simulink model "ThermalModel"  (R2021a)
settings: Solver=FixedStepAuto  StartTime=0.0  StopTime=28600  FixedStep=0.2  RelTol=1e-3
InitFcn:
  | %StartUp_VariableDeclaration;
undefined symbols (not defined in the file or in its folder): AxAlpha_Bottoms_Ambient, AxAlpha_Column_Ambient, AxAlpha_Head_Ambient, AxAlpha_Heater_Ambient, AxAlpha_Heater_Bottoms_Off, AxAlpha_Heater_Bottoms_On, AxAlpha_Heater_Inner_Outer, AxAlpha_Template, M_Water_Template, MxC_Bottoms, MxC_Column, MxC_Head, MxC_Heater_Inner, MxC_Heater_Outer, MxC_Template, T_init_Bottoms, T_init_Column, T_init_Head, T_init_Heater, T_init_Template, Temp_Water_Initial_Template
settings Model: OrderedModelArguments=off  Creator=Reinpold  LastModifiedBy=Reinpold

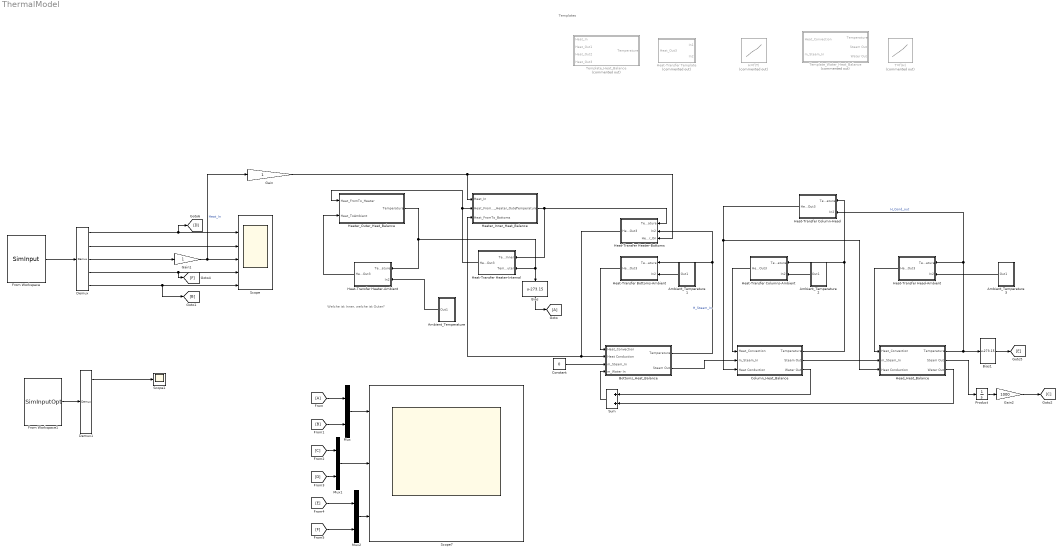
== system ThermalModel ==
  note: Welche ist Inner, welche ist Outer?
  note: Templates
  Ambient_Temperature : Subsystem
  Ambient_Temperature1 : Subsystem
  Ambient_Temperature2 : Subsystem
  Ambient_Temperature3 : Subsystem
  Bias : Bias  Bias=-273.15
  Bias1 : Bias  Bias=-273.15
  Bottoms_Heat_Balance : Subsystem
  Column_Heat_Balance : Subsystem
  Constant : Constant  Value=0
  Demux : Demux  Outputs=5
  Demux1 : Demux
  From Workspace : FromWorkspace  VariableName=SimInput
  From Workspace1 : FromWorkspace  VariableName=SimInputOpt  Interpolate=off  OutputAfterFinalValue=Holding final value
  Gain : Gain
  Gain1 : Gain
  Gain2 : Gain  Gain=1000
  H=f(T) : Lookup_n-D  Commented=on  NumberOfTableDimensions=1  BreakpointsForDimension1=|  Table=[0.10319804238124, 414.95098616583, 2675.58417423615, 2822.05078480503]  InternalRulePriority=Speed  RndMeth=Simplest  InputSameDT=on
      | [273.16, 372.15, 373.15, 446.15
      | ]
  Head_Heat_Balance : Subsystem
  Heat-Transfer Bottoms-Ambient : Subsystem
  Heat-Transfer Column-Head : Subsystem
  Heat-Transfer Columns-Ambient : Subsystem
  Heat-Transfer Head-Ambient : Subsystem
  Heat-Transfer Heater-Ambient : Subsystem
  Heat-Transfer Heater-Bottoms : Subsystem
  Heat-Transfer Heater-Internal : Subsystem
  Heat-Transfer Template : Subsystem  Commented=on
  Heater_Inner_Heat_Balance : Subsystem
  Heater_Outer_Heat_Balance : Subsystem
  Mux : Mux  Inputs=2
  Mux1 : Mux  Inputs=2
  Mux2 : Mux  Inputs=2
  Product : Integrator
  Scope : Scope  NumInputPorts=6
  Scope1 : Scope
  Scope7 : Scope  NumInputPorts=3
  Sum : Sum
  T=f(H) : Lookup_n-D  Commented=on  NumberOfTableDimensions=1  BreakpointsForDimension1=[0.10319804238124, 414.95098616583, 2675.58417423615, 2822.05078480503]  Table=[273.16, 372.15, 373.15, 446.15]  InternalRulePriority=Speed  RndMeth=Simplest  InputSameDT=on
  Template_Heat_Balance : Subsystem  Commented=on
  Template_Water_Heat_Balance : Subsystem  Commented=on
  wires:
  Gain1/1 -> Gain/1, Scope/4  "Heat_In"
  Ambient_Temperature/1(Out1) -> Heat-Transfer Heater-Ambient/2(In2)
  Heat-Transfer Heater-Ambient/1(Heat_Out3) -> Heater_Outer_Heat_Balance/2(Heat_ToAmbient)
  Heat-Transfer Heater-Bottoms/1(Heat_Out3) -> Bottoms_Heat_Balance/2(Heat Conduction), Heater_Inner_Heat_Balance/3(Heat_FromTo_Bottoms)
  Ambient_Temperature1/1(Out1) -> Heat-Transfer Bottoms-Ambient/2(In2)
  Heat-Transfer Bottoms-Ambient/1(Heat_Out3) -> Bottoms_Heat_Balance/1(Heat_Convection)
  Heat-Transfer Columns-Ambient/1(Heat_Out3) -> Column_Heat_Balance/1(Heat_Convection)
  Ambient_Temperature2/1(Out1) -> Heat-Transfer Columns-Ambient/2(In2)
  Heat-Transfer Head-Ambient/1(Heat_Out3) -> Head_Heat_Balance/1(Heat_Convection)
  Ambient_Temperature3/1(Out1) -> Heat-Transfer Head-Ambient/2(In2)
  Constant/1 -> Bottoms_Heat_Balance/3(m_Steam_In)
  Column_Heat_Balance/2(Steam Out) -> Head_Heat_Balance/2(m_Steam_In)
  Bottoms_Heat_Balance/2(Steam Out) -> Column_Heat_Balance/2(m_Steam_In)
  Product/1 -> Gain2/1
  Sum/1 -> Bottoms_Heat_Balance/4(m_Water In)
  Demux/2 -> Scope/3
  Demux/5 -> [B], Scope/6
  Bias1/1 -> [E]
  Column_Heat_Balance/3(Water Out) -> Sum/1
  Head_Heat_Balance/3(Water Out) -> Sum/2
  Head_Heat_Balance/2(Steam Out) -> Product/1
  From Workspace/1 -> Demux/1
  Gain2/1 -> [C]
  Heat-Transfer Column-Head/1(Heat_Out3) -> Head_Heat_Balance/3(Heat Conduction), Column_Heat_Balance/3(Heat Conduction)
  Column_Heat_Balance/1(Temperature) -> Heat-Transfer Columns-Ambient/1(Temperature), Heat-Transfer Column-Head/1(Temperature)
  Head_Heat_Balance/1(Temperature) -> Bias1/1, Heat-Transfer Column-Head/2(In2), Heat-Transfer Head-Ambient/1(Temperature)  "H_Cond_out"
  Heater_Inner_Heat_Balance/1(Temperature) -> Heat-Transfer Heater-Internal/1(Temperature_Inner), Heat-Transfer Heater-Bottoms/1(Temperature)
  Bottoms_Heat_Balance/1(Temperature) -> Heat-Transfer Heater-Bottoms/2(In2), Heat-Transfer Bottoms-Ambient/1(Temperature)  "H_Steam_In"
  Heater_Outer_Heat_Balance/1(Temperature) -> Bias/1, Heat-Transfer Heater-Internal/2(Temperature_Outer), Heat-Transfer Heater-Ambient/1(Temperature)
  Heat-Transfer Heater-Internal/1(Heat_Out3) -> Heater_Inner_Heat_Balance/2(Heat_FromTo_Heater_Outer), Heater_Outer_Heat_Balance/1(Heat_FromTo_Heater)
  [A] -> Mux/1
  [B] -> Mux/2
  [C] -> Mux1/1
  [D] -> Mux1/2
  [E] -> Mux2/1
  [F] -> Mux2/2
  Mux/1 -> Scope7/1
  Mux1/1 -> Scope7/2
  Mux2/1 -> Scope7/3
  Gain/1 -> Heat-Transfer Heater-Bottoms/3(Heater_On), Heater_Inner_Heat_Balance/1(Heat_In)
  Bias/1 -> [A]
  From Workspace1/1 -> Demux1/1
  Demux/1 -> Scope/2, [D]
  Demux/4 -> [F], Scope/5
  Demux/3 -> Gain1/1
  Demux1/1 -> Scope1/1

== system ThermalModel/Ambient_Temperature ==
  1-D Lookup Table : Lookup_n-D  NumberOfTableDimensions=1  BreakpointsForDimension1=[0,90*60,180*60,270*60,360*60]  Table=[21,23,23.5,24,24]  InternalRulePriority=Speed  RndMeth=Simplest  InputSameDT=on
  Bias2 : Bias  Bias=273.15
  Clock : Clock
  Out1 : Outport
  wires:
  1-D Lookup Table/1 -> Bias2/1
  Bias2/1 -> Out1/1
  Clock/1 -> 1-D Lookup Table/1

== system ThermalModel/Ambient_Temperature1 ==
  1-D Lookup Table : Lookup_n-D  NumberOfTableDimensions=1  BreakpointsForDimension1=[0,90*60,180*60,270*60,360*60]  Table=[21,23,23.5,24,24]  InternalRulePriority=Speed  RndMeth=Simplest  InputSameDT=on
  Bias2 : Bias  Bias=273.15
  Clock : Clock
  Out1 : Outport
  wires:
  1-D Lookup Table/1 -> Bias2/1
  Bias2/1 -> Out1/1
  Clock/1 -> 1-D Lookup Table/1

== system ThermalModel/Ambient_Temperature2 ==
  1-D Lookup Table : Lookup_n-D  NumberOfTableDimensions=1  BreakpointsForDimension1=[0,90*60,180*60,270*60,360*60]  Table=[21,23,23.5,24,24]  InternalRulePriority=Speed  RndMeth=Simplest  InputSameDT=on
  Bias2 : Bias  Bias=273.15
  Clock : Clock
  Out1 : Outport
  wires:
  1-D Lookup Table/1 -> Bias2/1
  Bias2/1 -> Out1/1
  Clock/1 -> 1-D Lookup Table/1

== system ThermalModel/Ambient_Temperature3 ==
  1-D Lookup Table : Lookup_n-D  NumberOfTableDimensions=1  BreakpointsForDimension1=[0,90*60,180*60,270*60,360*60]  Table=[21,23,23.5,24,24]  InternalRulePriority=Speed  RndMeth=Simplest  InputSameDT=on
  Bias2 : Bias  Bias=273.15
  Clock : Clock
  Out1 : Outport
  wires:
  1-D Lookup Table/1 -> Bias2/1
  Bias2/1 -> Out1/1
  Clock/1 -> 1-D Lookup Table/1

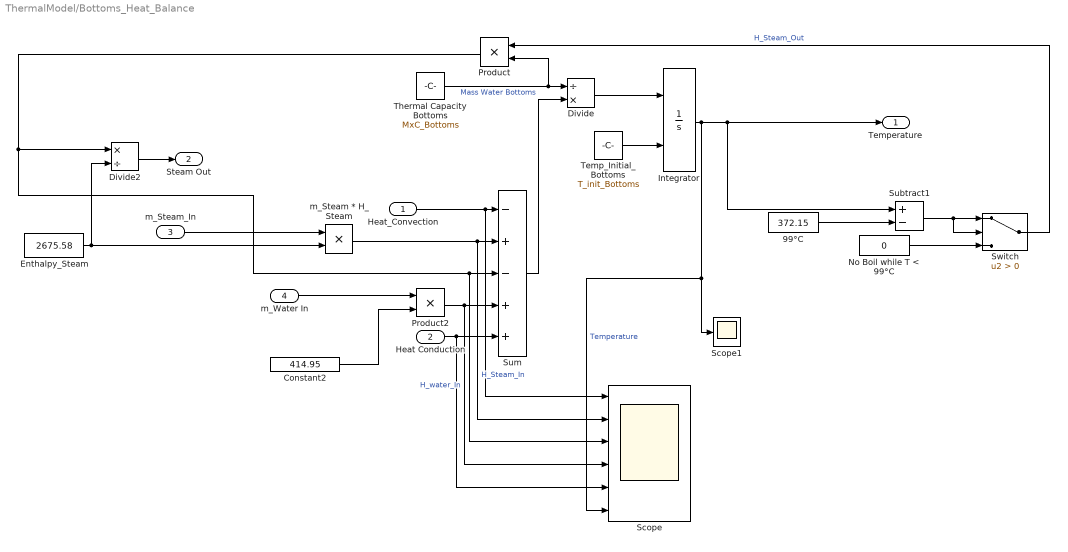
== system ThermalModel/Bottoms_Heat_Balance ==
  Heat_Convection : Inport
  Heat Conduction : Inport  Port=2
  m_Steam_In : Inport  Port=3
  m_Water In : Inport  Port=4
  " 99°C" : Constant  Value=372.15
  Constant2 : Constant  Value=414.95
  Divide : Product  Inputs=/*
  Divide2 : Product  Inputs=*/
  Enthalpy_Steam : Constant  Value=2675.58
  Integrator : Integrator  InitialConditionSource=external  UpperSaturationLimit=100
  No Boil while T < 99°C : Constant  Value=0
  Product : Product
  Product2 : Product
  Scope : Scope  NumInputPorts=6
  Scope1 : Scope
  Subtract1 : Sum  Inputs=+-
  Sum : Sum  Inputs=-+-++
  Switch : Switch  Criteria=u2 > Threshold
  Temp_Initial_Bottoms : Constant  Value=T_init_Bottoms
  Thermal Capacity Bottoms : Constant  Value=MxC_Bottoms
  m_Steam * H_Steam : Product
  Temperature : Outport
  Steam Out : Outport  Port=2
  wires:
  Switch/1 -> Product/1  "H_Steam_Out"
  Divide/1 -> Integrator/1
  Integrator/1 -> Scope1/1, Scope/6, Subtract1/1, Temperature/1  "Temperature"
  Thermal Capacity Bottoms/1 -> Product/2, Divide/1  "Mass Water Bottoms"
  Sum/1 -> Divide/2
  Heat_Convection/1 -> Scope/1, Sum/1
  m_Water In/1 -> Product2/1
  m_Steam_In/1 -> m_Steam * H_Steam/1
  m_Steam * H_Steam/1 -> Scope/2, Sum/2  "H_Steam_In"
  Enthalpy_Steam/1 -> Divide2/2, m_Steam * H_Steam/2
  Product2/1 -> Sum/4, Scope/4  "H_water_In"
  Temp_Initial_Bottoms/1 -> Integrator/2
  " 99°C"/1 -> Subtract1/2
  No Boil while T < 99°C/1 -> Switch/3
  Divide2/1 -> Steam Out/1
  Subtract1/1 -> Switch/2, Switch/1
  Product/1 -> Divide2/1, Scope/3, Sum/3
  Constant2/1 -> Product2/2
  Heat Conduction/1 -> Sum/5, Scope/5

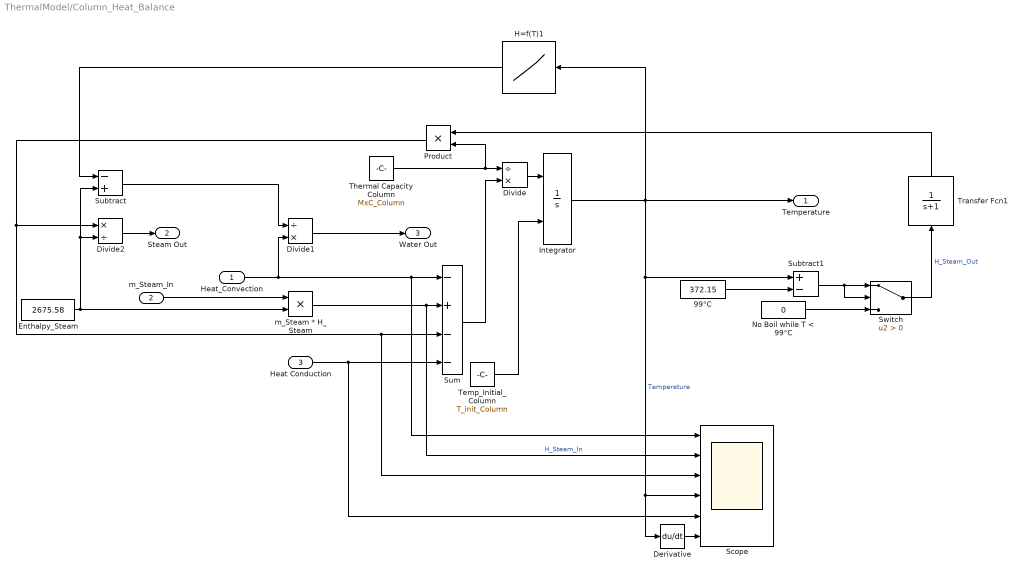
== system ThermalModel/Column_Heat_Balance ==
  Heat_Convection : Inport
  m_Steam_In : Inport  Port=2
  Heat Conduction : Inport  Port=3
  " 99°C" : Constant  Value=372.15
  Derivative : Derivative
  Divide : Product  Inputs=/*
  Divide1 : Product  Inputs=/*
  Divide2 : Product  Inputs=*/
  Enthalpy_Steam : Constant  Value=2675.58
  H=f(T)1 : Lookup_n-D  NumberOfTableDimensions=1  BreakpointsForDimension1=|  Table=[0.10319804238124, 414.95098616583, 2675.58417423615, 2822.05078480503]  InternalRulePriority=Speed  RndMeth=Simplest  InputSameDT=on
      | [273.16, 372.15, 373.15, 446.15
      | ]
  Integrator : Integrator  InitialConditionSource=external  UpperSaturationLimit=100
  No Boil while T < 99°C : Constant  Value=0
  Product : Product
  Scope : Scope  NumInputPorts=6
  Subtract : Sum  Inputs=-+
  Subtract1 : Sum  Inputs=+-
  Sum : Sum  Inputs=-+--
  Switch : Switch  Criteria=u2 > Threshold
  Temp_Initial_Column : Constant  Value=T_init_Column
  Thermal Capacity Column : Constant  Value=MxC_Column
  Transfer Fcn1 : TransferFcn  Denominator=[1 1]
  m_Steam * H_Steam : Product
  Temperature : Outport
  Steam Out : Outport  Port=2
  Water Out : Outport  Port=3
  wires:
  Switch/1 -> Transfer Fcn1/1  "H_Steam_Out"
  Thermal Capacity Column/1 -> Product/2, Divide/1
  Sum/1 -> Divide/2
  Heat_Convection/1 -> Divide1/2, Scope/1, Sum/1
  m_Steam_In/1 -> m_Steam * H_Steam/1
  m_Steam * H_Steam/1 -> Scope/2, Sum/2  "H_Steam_In"
  Enthalpy_Steam/1 -> Subtract/2, Divide2/2, m_Steam * H_Steam/2
  Temp_Initial_Column/1 -> Integrator/2
  " 99°C"/1 -> Subtract1/2
  No Boil while T < 99°C/1 -> Switch/3
  Divide2/1 -> Steam Out/1
  Subtract1/1 -> Switch/2, Switch/1
  Product/1 -> Divide2/1, Scope/3, Sum/3
  Subtract/1 -> Divide1/1
  Divide1/1 -> Water Out/1
  Divide/1 -> Integrator/1
  H=f(T)1/1 -> Subtract/1
  Heat Conduction/1 -> Scope/5, Sum/4
  Transfer Fcn1/1 -> Product/1
  Integrator/1 -> H=f(T)1/1, Temperature/1, Derivative/1, Scope/4, Subtract1/1  "Temperature"
  Derivative/1 -> Scope/6

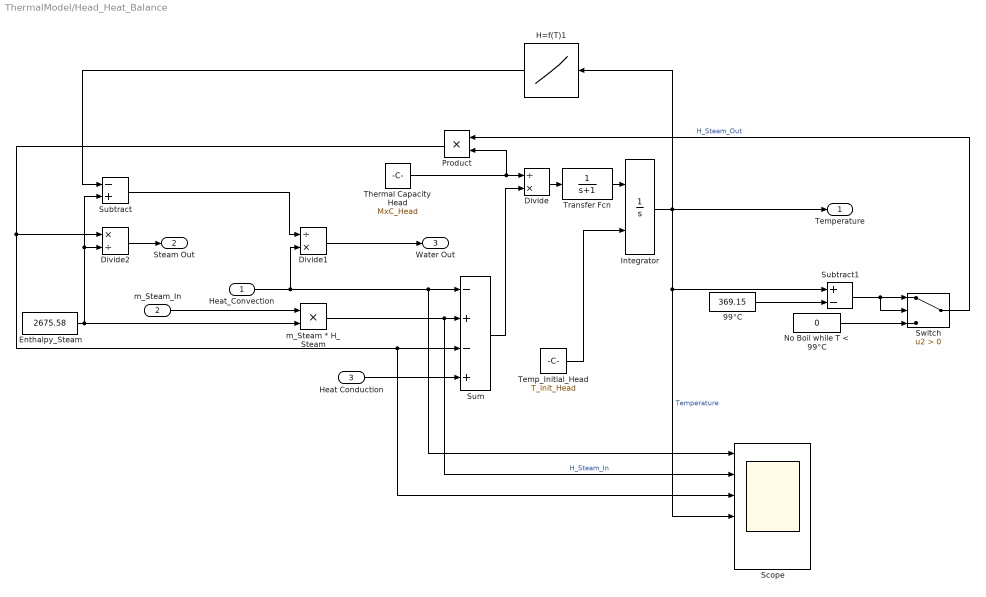
== system ThermalModel/Head_Heat_Balance ==
  Heat_Convection : Inport
  m_Steam_In : Inport  Port=2
  Heat Conduction : Inport  Port=3
  " 99°C" : Constant  Value=369.15
  Divide : Product  Inputs=/*
  Divide1 : Product  Inputs=/*
  Divide2 : Product  Inputs=*/
  Enthalpy_Steam : Constant  Value=2675.58
  H=f(T)1 : Lookup_n-D  NumberOfTableDimensions=1  BreakpointsForDimension1=|  Table=[0.10319804238124, 414.95098616583, 2675.58417423615, 2822.05078480503]  InternalRulePriority=Speed  RndMeth=Simplest  InputSameDT=on
      | [273.16, 372.15, 373.15, 446.15
      | ]
  Integrator : Integrator  InitialConditionSource=external  UpperSaturationLimit=100
  No Boil while T < 99°C : Constant  Value=0
  Product : Product
  Scope : Scope  NumInputPorts=6
  Subtract : Sum  Inputs=-+
  Subtract1 : Sum  Inputs=+-
  Sum : Sum  Inputs=-+-+
  Switch : Switch  Criteria=u2 > Threshold
  Temp_Initial_Head : Constant  Value=T_init_Head
  Thermal Capacity Head : Constant  Value=MxC_Head
  Transfer Fcn : TransferFcn  Denominator=[1 1]
  m_Steam * H_Steam : Product
  Temperature : Outport
  Steam Out : Outport  Port=2
  Water Out : Outport  Port=3
  wires:
  Switch/1 -> Product/1  "H_Steam_Out"
  Divide/1 -> Transfer Fcn/1
  Integrator/1 -> H=f(T)1/1, Temperature/1, Scope/4, Subtract1/1  "Temperature"
  Thermal Capacity Head/1 -> Product/2, Divide/1
  Sum/1 -> Divide/2
  Heat_Convection/1 -> Divide1/2, Scope/1, Sum/1
  m_Steam_In/1 -> m_Steam * H_Steam/1
  m_Steam * H_Steam/1 -> Scope/2, Sum/2  "H_Steam_In"
  Enthalpy_Steam/1 -> Subtract/2, Divide2/2, m_Steam * H_Steam/2
  Temp_Initial_Head/1 -> Integrator/2
  " 99°C"/1 -> Subtract1/2
  No Boil while T < 99°C/1 -> Switch/3
  Divide2/1 -> Steam Out/1
  Subtract1/1 -> Switch/2, Switch/1
  Product/1 -> Divide2/1, Scope/3, Sum/3
  Subtract/1 -> Divide1/1
  Divide1/1 -> Water Out/1
  Transfer Fcn/1 -> Integrator/1
  H=f(T)1/1 -> Subtract/1
  Heat Conduction/1 -> Sum/4

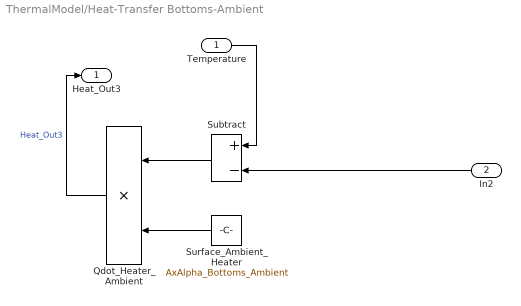
== system ThermalModel/Heat-Transfer Bottoms-Ambient ==
  Temperature : Inport
  In2 : Inport  Port=2
  Qdot_Heater_Ambient : Product
  Subtract : Sum  Inputs=+-
  Surface_Ambient_Heater : Constant  Value=AxAlpha_Bottoms_Ambient
  Heat_Out3 : Outport
  wires:
  Subtract/1 -> Qdot_Heater_Ambient/1
  Surface_Ambient_Heater/1 -> Qdot_Heater_Ambient/2
  In2/1 -> Subtract/2
  Qdot_Heater_Ambient/1 -> Heat_Out3/1  "Heat_Out3"
  Temperature/1 -> Subtract/1

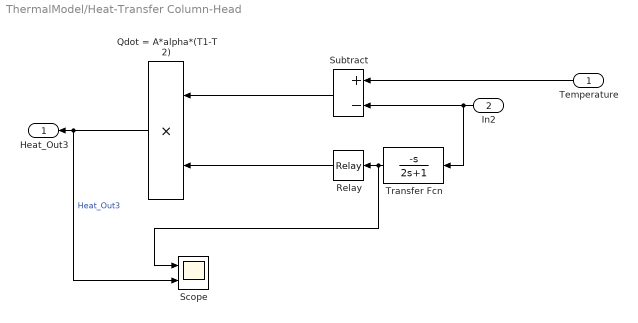
== system ThermalModel/Heat-Transfer Column-Head ==
  Temperature : Inport
  In2 : Inport  Port=2
  Qdot = A*alpha*(T1-T2) : Product
  Relay : Relay  OnSwitchValue=0.03  OffSwitchValue=-0.005  OnOutputValue=AxAlpha_Column_Head
  Scope : Scope  NumInputPorts=2
  Subtract : Sum  Inputs=+-
  Transfer Fcn : TransferFcn  Numerator=[-1 0]  Denominator=[2 1]
  Heat_Out3 : Outport
  wires:
  Subtract/1 -> Qdot = A*alpha*(T1-T2)/1
  In2/1 -> Transfer Fcn/1, Subtract/2
  Qdot = A*alpha*(T1-T2)/1 -> Scope/2, Heat_Out3/1  "Heat_Out3"
  Temperature/1 -> Subtract/1
  Transfer Fcn/1 -> Scope/1, Relay/1
  Relay/1 -> Qdot = A*alpha*(T1-T2)/2

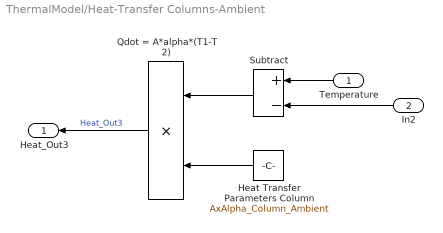
== system ThermalModel/Heat-Transfer Columns-Ambient ==
  Temperature : Inport
  In2 : Inport  Port=2
  Heat Transfer Parameters Column : Constant  Value=AxAlpha_Column_Ambient
  Qdot = A*alpha*(T1-T2) : Product
  Subtract : Sum  Inputs=+-
  Heat_Out3 : Outport
  wires:
  Subtract/1 -> Qdot = A*alpha*(T1-T2)/1
  Heat Transfer Parameters Column/1 -> Qdot = A*alpha*(T1-T2)/2
  In2/1 -> Subtract/2
  Qdot = A*alpha*(T1-T2)/1 -> Heat_Out3/1  "Heat_Out3"
  Temperature/1 -> Subtract/1

== system ThermalModel/Heat-Transfer Head-Ambient ==
  Temperature : Inport
  In2 : Inport  Port=2
  Heat Transfer Parameters_Head : Constant  Value=AxAlpha_Head_Ambient
  Qdot = A*alpha*(T1-T2) : Product
  Subtract : Sum  Inputs=+-
  Heat_Out3 : Outport
  wires:
  Subtract/1 -> Qdot = A*alpha*(T1-T2)/1
  Heat Transfer Parameters_Head/1 -> Qdot = A*alpha*(T1-T2)/2
  In2/1 -> Subtract/2
  Qdot = A*alpha*(T1-T2)/1 -> Heat_Out3/1  "Heat_Out3"
  Temperature/1 -> Subtract/1

== system ThermalModel/Heat-Transfer Heater-Ambient ==
  Temperature : Inport
  In2 : Inport  Port=2
  Heat Transfer Parameters Heater_Ambeint : Constant  Value=AxAlpha_Heater_Ambient
  Qdot_Heater_Ambient : Product
  Subtract : Sum  Inputs=+-
  Heat_Out3 : Outport
  wires:
  Subtract/1 -> Qdot_Heater_Ambient/1
  Heat Transfer Parameters Heater_Ambeint/1 -> Qdot_Heater_Ambient/2
  In2/1 -> Subtract/2
  Qdot_Heater_Ambient/1 -> Heat_Out3/1  "Heat_Out3"
  Temperature/1 -> Subtract/1

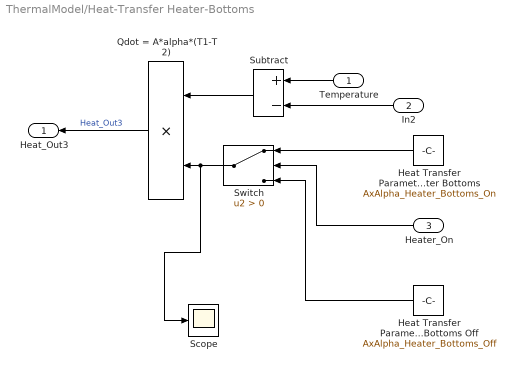
== system ThermalModel/Heat-Transfer Heater-Bottoms ==
  Temperature : Inport
  In2 : Inport  Port=2
  Heater_On : Inport  Port=3
  Heat Transfer Parameters Heater Bottoms : Constant  Value=AxAlpha_Heater_Bottoms_On
  Heat Transfer Parameters Heater Bottoms Off : Constant  Value=AxAlpha_Heater_Bottoms_Off
  Qdot = A*alpha*(T1-T2) : Product
  Scope : Scope
  Subtract : Sum  Inputs=+-
  Switch : Switch  Criteria=u2 > Threshold
  Heat_Out3 : Outport
  wires:
  Subtract/1 -> Qdot = A*alpha*(T1-T2)/1
  Heat Transfer Parameters Heater Bottoms/1 -> Switch/1
  In2/1 -> Subtract/2
  Qdot = A*alpha*(T1-T2)/1 -> Heat_Out3/1  "Heat_Out3"
  Temperature/1 -> Subtract/1
  Heat Transfer Parameters Heater Bottoms Off/1 -> Switch/3
  Heater_On/1 -> Switch/2
  Switch/1 -> Scope/1, Qdot = A*alpha*(T1-T2)/2

== system ThermalModel/Heat-Transfer Heater-Internal ==
  Temperature_Inner : Inport
  Temperature_Outer : Inport  Port=2
  Heat Transfer Parameters Heater Bottoms : Constant  Value=AxAlpha_Heater_Inner_Outer
  Qdot = A*alpha*(T1-T2) : Product
  Subtract : Sum  Inputs=+-
  Heat_Out3 : Outport
  wires:
  Subtract/1 -> Qdot = A*alpha*(T1-T2)/1
  Heat Transfer Parameters Heater Bottoms/1 -> Qdot = A*alpha*(T1-T2)/2
  Temperature_Outer/1 -> Subtract/2
  Qdot = A*alpha*(T1-T2)/1 -> Heat_Out3/1  "Heat_Out3"
  Temperature_Inner/1 -> Subtract/1

== system ThermalModel/Heat-Transfer Template ==
  In1 : Inport
  In2 : Inport  Port=2
  Heat Transfer Parameters_Template : Constant  Value=AxAlpha_Template
  Qdot = A*alpha*(T1-T2) : Product
  Subtract : Sum  Inputs=+-
  Heat_Out3 : Outport
  wires:
  Subtract/1 -> Qdot = A*alpha*(T1-T2)/1
  Heat Transfer Parameters_Template/1 -> Qdot = A*alpha*(T1-T2)/2
  In2/1 -> Subtract/2
  Qdot = A*alpha*(T1-T2)/1 -> Heat_Out3/1  "Heat_Out3"
  In1/1 -> Subtract/1

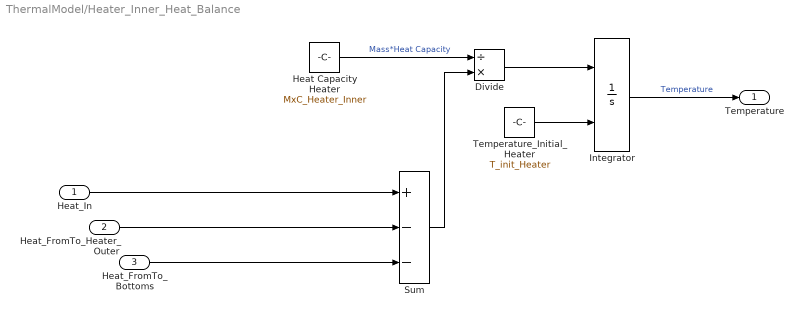
== system ThermalModel/Heater_Inner_Heat_Balance ==
  Heat_In : Inport
  Heat_FromTo_Heater_Outer : Inport  Port=2
  Heat_FromTo_Bottoms : Inport  Port=3
  Divide : Product  Inputs=/*
  Heat Capacity Heater : Constant  Value=MxC_Heater_Inner
  Integrator : Integrator  InitialConditionSource=external
  Sum : Sum  Inputs=+--
  Temperature_Initial_Heater : Constant  Value=T_init_Heater
  Temperature : Outport
  wires:
  Heat_FromTo_Bottoms/1 -> Sum/3
  Divide/1 -> Integrator/1
  Integrator/1 -> Temperature/1  "Temperature"
  Temperature_Initial_Heater/1 -> Integrator/2
  Heat Capacity Heater/1 -> Divide/1  "Mass*Heat Capacity"
  Sum/1 -> Divide/2
  Heat_In/1 -> Sum/1
  Heat_FromTo_Heater_Outer/1 -> Sum/2

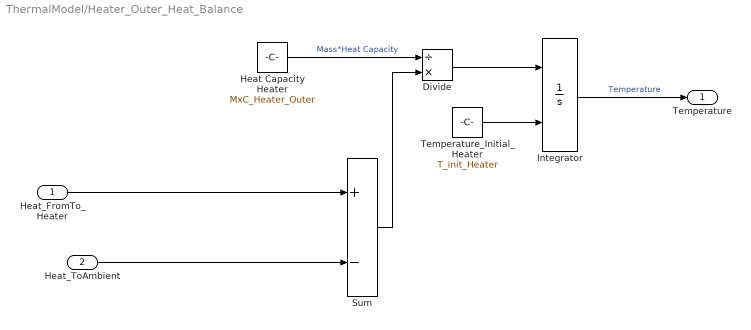
== system ThermalModel/Heater_Outer_Heat_Balance ==
  Heat_FromTo_Heater : Inport
  Heat_ToAmbient : Inport  Port=2
  Divide : Product  Inputs=/*
  Heat Capacity Heater : Constant  Value=MxC_Heater_Outer
  Integrator : Integrator  InitialConditionSource=external
  Sum : Sum  Inputs=+-
  Temperature_Initial_Heater : Constant  Value=T_init_Heater
  Temperature : Outport
  wires:
  Heat_ToAmbient/1 -> Sum/2
  Divide/1 -> Integrator/1
  Integrator/1 -> Temperature/1  "Temperature"
  Temperature_Initial_Heater/1 -> Integrator/2
  Heat Capacity Heater/1 -> Divide/1  "Mass*Heat Capacity"
  Sum/1 -> Divide/2
  Heat_FromTo_Heater/1 -> Sum/1

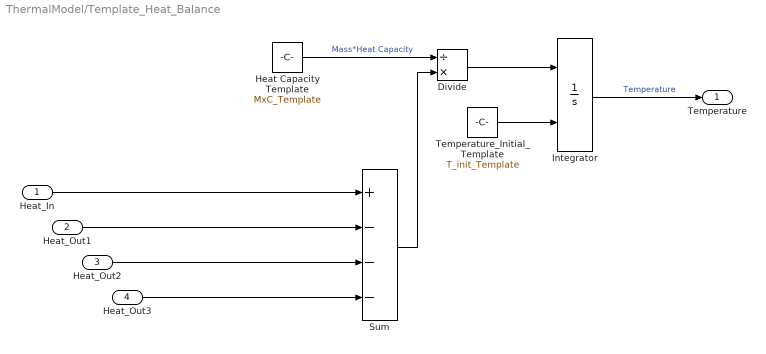
== system ThermalModel/Template_Heat_Balance ==
  Heat_In : Inport
  Heat_Out1 : Inport  Port=2
  Heat_Out2 : Inport  Port=3
  Heat_Out3 : Inport  Port=4
  Divide : Product  Inputs=/*
  Heat Capacity Template : Constant  Value=MxC_Template
  Integrator : Integrator  InitialConditionSource=external
  Sum : Sum  Inputs=+---
  Temperature_Initial_Template : Constant  Value=T_init_Template
  Temperature : Outport
  wires:
  Heat_Out2/1 -> Sum/3
  Divide/1 -> Integrator/1
  Integrator/1 -> Temperature/1  "Temperature"
  Temperature_Initial_Template/1 -> Integrator/2
  Heat Capacity Template/1 -> Divide/1  "Mass*Heat Capacity"
  Sum/1 -> Divide/2
  Heat_In/1 -> Sum/1
  Heat_Out3/1 -> Sum/4
  Heat_Out1/1 -> Sum/2

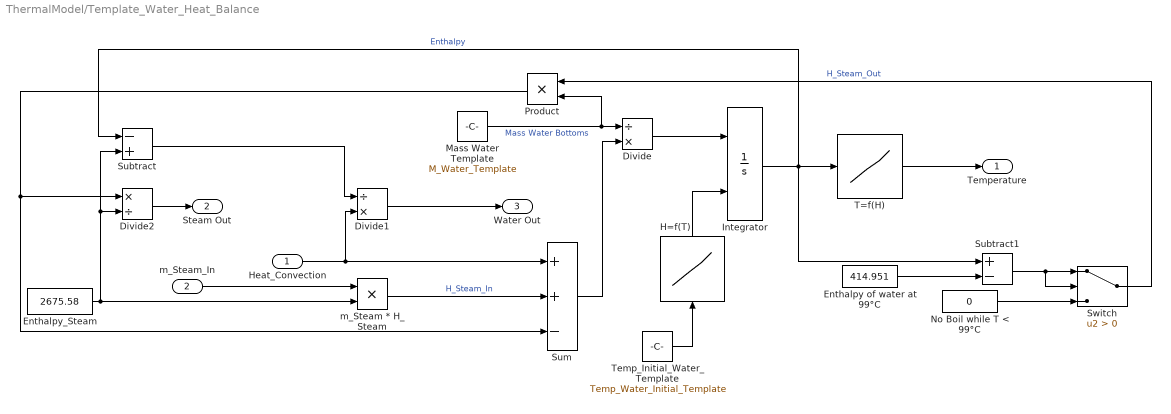
== system ThermalModel/Template_Water_Heat_Balance ==
  Heat_Convection : Inport
  m_Steam_In : Inport  Port=2
  Divide : Product  Inputs=/*
  Divide1 : Product  Inputs=/*
  Divide2 : Product  Inputs=*/
  Enthalpy of water at 99°C : Constant  Value=414.951
  Enthalpy_Steam : Constant  Value=2675.58
  H=f(T) : Lookup_n-D  NumberOfTableDimensions=1  BreakpointsForDimension1=|  Table=[0.10319804238124, 414.95098616583, 2675.58417423615, 2822.05078480503]  InternalRulePriority=Speed  RndMeth=Simplest  InputSameDT=on
      | [273.16, 372.15, 373.15, 446.15
      | ]
  Integrator : Integrator  InitialConditionSource=external  UpperSaturationLimit=100
  Mass Water Template : Constant  Value=M_Water_Template
  No Boil while T < 99°C : Constant  Value=0
  Product : Product
  Subtract : Sum  Inputs=-+
  Subtract1 : Sum  Inputs=+-
  Sum : Sum  Inputs=++-
  Switch : Switch  Criteria=u2 > Threshold
  T=f(H) : Lookup_n-D  NumberOfTableDimensions=1  BreakpointsForDimension1=[0.10319804238124, 414.95098616583, 2675.58417423615, 2822.05078480503]  Table=[273.16, 372.15, 373.15, 446.15]  InternalRulePriority=Speed  RndMeth=Simplest  InputSameDT=on
  Temp_Initial_Water_Template : Constant  Value=Temp_Water_Initial_Template
  m_Steam * H_Steam : Product
  Temperature : Outport
  Steam Out : Outport  Port=2
  Water Out : Outport  Port=3
  wires:
  Switch/1 -> Product/1  "H_Steam_Out"
  Divide/1 -> Integrator/1
  Integrator/1 -> Subtract/1, Subtract1/1, T=f(H)/1  "Enthalpy"
  Temp_Initial_Water_Template/1 -> H=f(T)/1
  Mass Water Template/1 -> Product/2, Divide/1  "Mass Water Bottoms"
  Sum/1 -> Divide/2
  Heat_Convection/1 -> Divide1/2, Sum/1
  m_Steam_In/1 -> m_Steam * H_Steam/1
  T=f(H)/1 -> Temperature/1
  m_Steam * H_Steam/1 -> Sum/2  "H_Steam_In"
  Enthalpy_Steam/1 -> Subtract/2, Divide2/2, m_Steam * H_Steam/2
  H=f(T)/1 -> Integrator/2
  Enthalpy of water at 99°C/1 -> Subtract1/2
  No Boil while T < 99°C/1 -> Switch/3
  Divide2/1 -> Steam Out/1
  Subtract1/1 -> Switch/2, Switch/1
  Product/1 -> Divide2/1, Sum/3
  Subtract/1 -> Divide1/1
  Divide1/1 -> Water Out/1
